simulink subsystem "pm_theta_r_observer_backEMF"  (R2022b)
settings: Solver=VariableStepAuto  StartTime=0.0  StopTime=10.0  RelTol=1e-3
values from neighbouring files (symbols this model uses):
  Ke = 100000    [pm_params_sensorless.m]
  Ki = 10    [pm_params_sensorless.m]
  Lamda_f = 0.123    [pm_params_sensorless.m]
  Ls = 0.085    [im_params_sensorless.m]    (also in pm_params_sensorless.m = 0.0091)
  pole = 4    [im_params_sensorless.m]    (also in pm_params_sensorless.m)
  Rs = 0.8    [im_params_sensorless.m]    (also in pm_params_sensorless.m = 1.2)
settings Model: Creator=jack  LastModifiedBy=jack

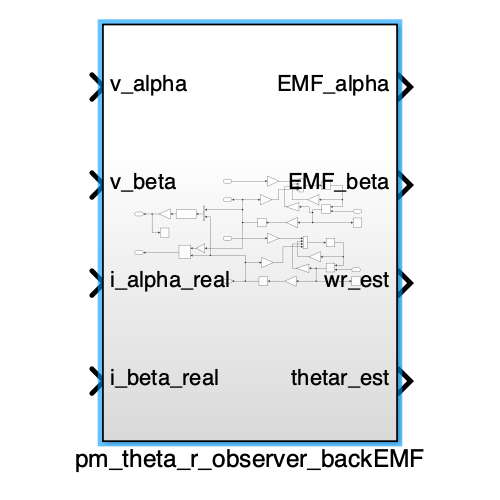
[thumbnail: Simulink's stored preview of the top-level diagram]
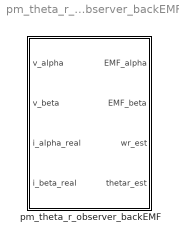
== system pm_theta_r_observer_backEMF ==
  pm_theta_r_observer_backEMF : Subsystem

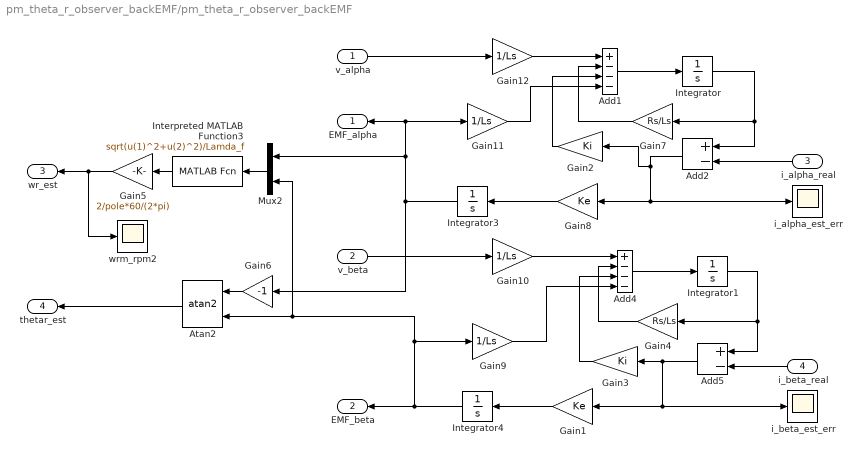
== system pm_theta_r_observer_backEMF/pm_theta_r_observer_backEMF ==
  v_alpha : Inport
  v_beta : Inport  Port=2
  i_alpha_real : Inport  Port=3
  i_beta_real : Inport  Port=4
  Add1 : Sum  Inputs=+---
  Add2 : Sum  Inputs=+-
  Add4 : Sum  Inputs=+---
  Add5 : Sum  Inputs=+-
  Atan2 : Trigonometry  Operator=atan2
  Gain1 : Gain  Gain=Ke
  Gain{9..12} (4 alike) : Gain  Gain=1/Ls
  Gain2 : Gain  Gain=Ki
  Gain3 : Gain  Gain=Ki
  Gain4 : Gain  Gain=Rs/Ls
  Gain5 : Gain  Gain=2/pole*60/(2*pi)
  Gain6 : Gain  Gain=-1
  Gain7 : Gain  Gain=Rs/Ls
  Gain8 : Gain  Gain=Ke
  Integrator{,1,3..4} (4 alike) : Integrator
  Interpreted MATLAB Function3 : MATLABFcn  MATLABFcn=sqrt(u(1)^2+u(2)^2)/Lamda_f
  Mux2 : Mux  Inputs=2
  i_alpha_est_err : Scope
  i_beta_est_err : Scope
  wrm_rpm2 : Scope
  EMF_alpha : Outport
  EMF_beta : Outport  Port=2
  wr_est : Outport  Port=3
  thetar_est : Outport  Port=4
  wires:
  Integrator4/1 -> Mux2/2, Atan2/2, Gain9/1, EMF_beta/1
  Integrator1/1 -> Gain4/1, Add5/1
  Gain4/1 -> Add4/2
  Add2/1 -> i_alpha_est_err/1, Gain8/1, Gain2/1
  Add4/1 -> Integrator1/1
  Integrator3/1 -> Mux2/1, Gain11/1, EMF_alpha/1, Gain6/1
  i_beta_real/1 -> Add5/2
  Gain9/1 -> Add4/4
  Add1/1 -> Integrator/1
  Mux2/1 -> Interpreted MATLAB Function3/1
  v_alpha/1 -> Gain12/1
  Gain3/1 -> Add4/3
  Gain5/1 -> wr_est/1, wrm_rpm2/1
  i_alpha_real/1 -> Add2/2
  Gain10/1 -> Add4/1
  Atan2/1 -> thetar_est/1
  Interpreted MATLAB Function3/1 -> Gain5/1
  Add5/1 -> Gain3/1, Gain1/1, i_beta_est_err/1
  Gain1/1 -> Integrator4/1
  Integrator/1 -> Gain7/1, Add2/1
  v_beta/1 -> Gain10/1
  Gain12/1 -> Add1/1
  Gain6/1 -> Atan2/1
  Gain11/1 -> Add1/4
  Gain8/1 -> Integrator3/1
  Gain7/1 -> Add1/2
  Gain2/1 -> Add1/3
